simulink model "DC_motor_subsystem_lib"  (Simulink 8.7)
settings: Solver=VariableStepAuto  StartTime=0.0  StopTime=10.0  RelTol=1e-3
settings Model: Creator=Shinelon  LastModifiedBy=Shinelon
settings DataIOCC: LimitDataPoints=off  SaveFormat=Dataset
settings DebuggingCC: UnderspecifiedInitializationDetection=Simplified  MergeDetectMultiDrivingBlocksExec=error
settings HardwareCC: ProdBitPerPointer=64  ProdLargestAtomicFloat=Float  ProdIntDivRoundTo=Zero  ProdEndianess=LittleEndian  ProdWordSize=64  ProdHWDeviceType=Intel->x86-64 (Windows64)
settings ModelReferenceCC: PropagateSignalLabelsOutOfModel=on
settings ConfigComp: CovModelRefEnable=off

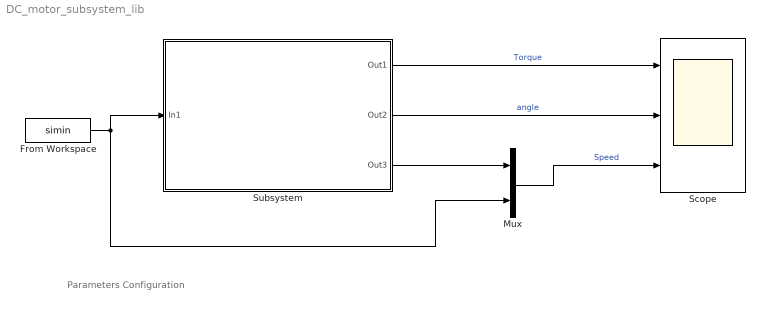
== system DC_motor_subsystem_lib ==
  note: Parameters
      | Configuration
  From Workspace : FromWorkspace  VariableName=simin  SampleTime=0
  Mux : Mux  Inputs=2
  Scope : Scope  NumInputPorts=3
  Subsystem : Subsystem  mask(DC motor subsystem){R=0, L=0, Km=0, Kf=0, Kemf=0, J=0}
      mask prompts: R "Resistor"; L "Inductor"; Km "Torque Constant"; Kf "Viscous Friction Constant"; Kemf "Back EMF Votage Constant"; J "Inertial Load"
      mask help:
      | This is a DC motor subsystem
      | Input : Control Signal
      | Output : Motor Rate
      mask init:
      | R=2;
      | L=0.5;
      | Km=0.1;
      | Kemf=0.1;
      | Kf=0.2;
      | J=0.02;
      mask Display:
      | color('red');port_label('input',1,'Control Signal');
      | color('red');port_label('output',1,'Torque');
      | color('red');port_label('output',2,'Angle');
      | color('red');port_label('output',3,'Speed');
      | image(imread('E:\simulink model\DC motor model\timg.jpg'))
  wires:
  From Workspace/1 -> Mux/2, Subsystem/1(In1)
  Mux/1 -> Scope/3  "Speed"
  Subsystem/1(Out1) -> Scope/1  "Torque"
  Subsystem/2(Out2) -> Scope/2  "angle"
  Subsystem/3(Out3) -> Mux/1

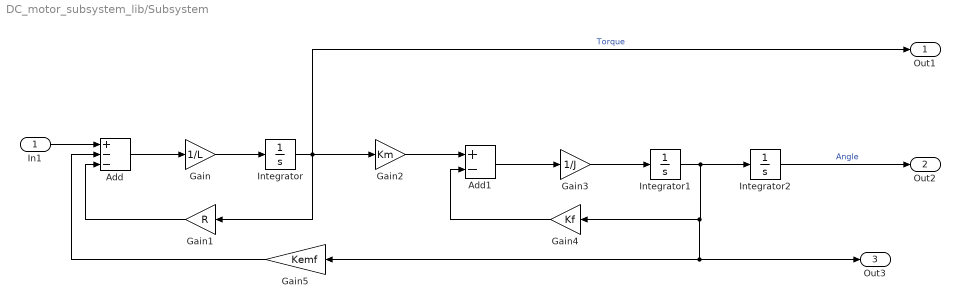
== system DC_motor_subsystem_lib/Subsystem ==
  In1 : Inport
  Add : Sum  Inputs=+--
  Add1 : Sum  Inputs=+-
  Gain : Gain  Gain=1/L
  Gain1 : Gain  Gain=R
  Gain2 : Gain  Gain=Km
  Gain3 : Gain  Gain=1/J
  Gain4 : Gain  Gain=Kf
  Gain5 : Gain  Gain=Kemf
  Integrator : Integrator
  Integrator1 : Integrator
  Integrator2 : Integrator
  Out1 : Outport
  Out2 : Outport  Port=2
  Out3 : Outport  Port=3
  wires:
  Gain5/1 -> Add/2
  Integrator/1 -> Out1/1, Gain2/1, Gain1/1  "Torque"
  Integrator2/1 -> Out2/1  "Angle"
  Add/1 -> Gain/1
  Gain/1 -> Integrator/1
  Gain1/1 -> Add/3
  Gain2/1 -> Add1/1
  Add1/1 -> Gain3/1
  Gain3/1 -> Integrator1/1
  Integrator1/1 -> Integrator2/1, Out3/1, Gain5/1, Gain4/1
  Gain4/1 -> Add1/2
  In1/1 -> Add/1
